simulink model "RR"  (R2015b)
settings: Solver=VariableStepAuto  StartTime=0.0  StopTime=10.0  RelTol=1e-3
undefined symbols (not defined in the file): alpha, b, beta, c, Csrr, gama, Ksrr, Kurr, m, Ps, S, tao
settings Model: Creator=Guest  LastModifiedBy=Guest

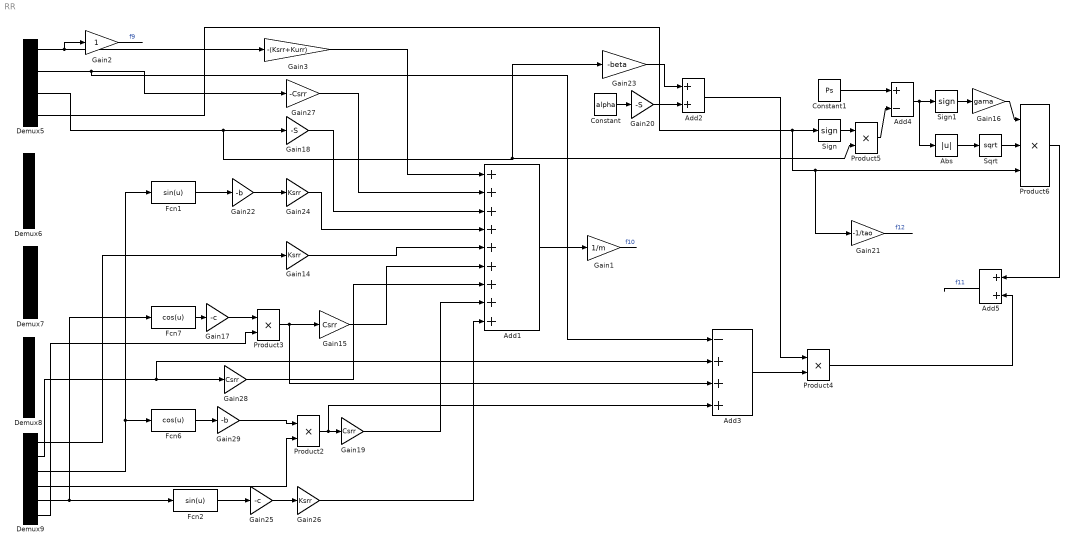
== system RR ==
  Abs : Abs
  Add1 : Sum  Inputs=+++++++++
  Add2 : Sum
  Add3 : Sum  Inputs=-+++
  Add4 : Sum  Inputs=+-
  Add5 : Sum
  Constant : Constant  Value=alpha
  Constant1 : Constant  Value=Ps
  Demux{5..8} (4 alike) : Demux
  Demux9 : Demux  Outputs=6
  Fcn1 : Fcn  Expr=sin(u)
  Fcn2 : Fcn  Expr=sin(u)
  Fcn6 : Fcn  Expr=cos(u)
  Fcn7 : Fcn  Expr=cos(u)
  Gain1 : Gain  Gain=1/m
  Gain14 : Gain  Gain=Ksrr
  Gain15 : Gain  Gain=Csrr
  Gain16 : Gain  Gain=gama
  Gain17 : Gain  Gain=-c
  Gain18 : Gain  Gain=-S
  Gain19 : Gain  Gain=Csrr
  Gain2 : Gain
  Gain20 : Gain  Gain=-S
  Gain21 : Gain  Gain=-1/tao
  Gain22 : Gain  Gain=-b
  Gain23 : Gain  Gain=-beta
  Gain24 : Gain  Gain=Ksrr
  Gain25 : Gain  Gain=-c
  Gain26 : Gain  Gain=Ksrr
  Gain27 : Gain  Gain=-Csrr
  Gain28 : Gain  Gain=Csrr
  Gain29 : Gain  Gain=-b
  Gain3 : Gain  Gain=-(Ksrr+Kurr)
  Product{2..5} (4 alike) : Product
  Product6 : Product  Inputs=3
  Sign : Signum
  Sign1 : Signum
  Sqrt : Sqrt  SaturateOnIntegerOverflow=on
  wires:
  Demux5/1 -> Gain2/1, Gain3/1
  Demux9/1 -> Gain14/1
  Demux9/3 -> Fcn1/1, Fcn6/1
  Fcn1/1 -> Gain22/1
  Gain22/1 -> Gain24/1
  Demux9/5 -> Fcn7/1, Fcn2/1
  Fcn2/1 -> Gain25/1
  Gain25/1 -> Gain26/1
  Demux5/2 -> Add3/1, Gain27/1
  Demux9/2 -> Add3/2, Gain28/1
  Fcn6/1 -> Gain29/1
  Gain29/1 -> Product2/1
  Demux9/4 -> Product2/2
  Fcn7/1 -> Gain17/1
  Demux9/6 -> Product3/2
  Gain17/1 -> Product3/1
  Demux5/3 -> Gain23/1, Product5/2, Gain18/1
  Gain3/1 -> Add1/1
  Gain27/1 -> Add1/2
  Gain18/1 -> Add1/3
  Gain24/1 -> Add1/4
  Gain14/1 -> Add1/5
  Product3/1 -> Add3/3, Gain15/1
  Gain28/1 -> Add1/7
  Product2/1 -> Add3/4, Gain19/1
  Gain26/1 -> Add1/9
  Constant/1 -> Gain20/1
  Gain23/1 -> Add2/1
  Gain20/1 -> Add2/2
  Gain19/1 -> Add1/8
  Gain15/1 -> Add1/6
  Add3/1 -> Product4/2
  Add2/1 -> Product4/1
  Demux5/4 -> Gain21/1, Product6/3, Sign/1
  Sign/1 -> Product5/1
  Constant1/1 -> Add4/1
  Product5/1 -> Add4/2
  Add4/1 -> Abs/1, Sign1/1
  Sign1/1 -> Gain16/1
  Abs/1 -> Sqrt/1
  Gain16/1 -> Product6/1
  Sqrt/1 -> Product6/2
  Product4/1 -> Add5/2
  Add1/1 -> Gain1/1
  Gain2/1 -> ?  "f9"
  Gain1/1 -> ?  "f10"
  Product6/1 -> Add5/1
  Add5/1 -> ?  "f11"
  Gain21/1 -> ?  "f12"
